simulink model "toneSelector"  (R2017b)
settings: Solver=VariableStepAuto  StartTime=0.0  StopTime=35  RelTol=1e-3
undefined symbols (not defined in the file): Ts
libraries: simulink x3, dspsnks4 x1
settings Model: Creator=pipe  LastModifiedBy=pipe

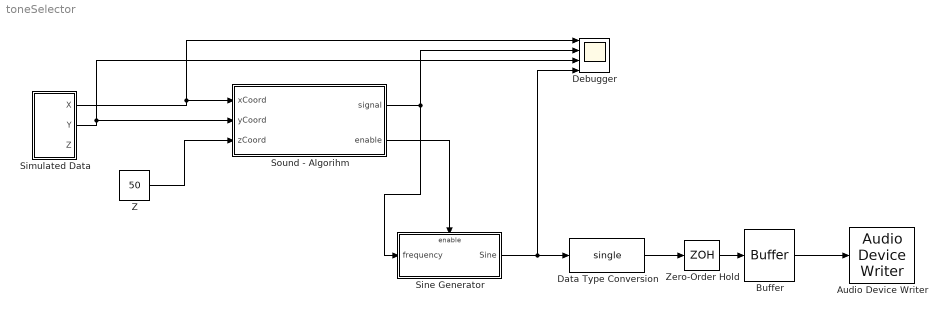
== system toneSelector ==
  Audio Device Writer : dspsnks4/Audio Device Writer  Driver=DirectSound  Device=Default  InheritSampleRate=on  SampleRate=40000  BitDepth=16-bit integer  BufferSize=4096  NumBuffers=10  DefaultOutputChannelMapping=on  OutputChannelMapping=1:2  OutputNumUnderrunSamples=off  DriverIdx=1  DeviceWarnFlag=''
  Buffer : Buffer  N=128  OutputFrames=off
  Data Type Conversion : DataTypeConversion  OutDataTypeStr=single
  "Debugger " : Scope  NumInputPorts=4
  Simulated Data : Subsystem
  Sine Generator : Subsystem  TreatAsAtomicUnit=on
  "Sound - Algorihm " : MATLAB Function  TreatAsAtomicUnit=on
  "Z " : Constant  Value=50  SampleTime=-1
  Zero-Order Hold : ZeroOrderHold  SampleTime=1/10000
  wires:
  "Sound - Algorihm "/1(signal) -> Sine Generator/1("frequency "), "Debugger "/2
  "Z "/1 -> "Sound - Algorihm "/3(zCoord)
  Simulated Data/1("X ") -> "Debugger "/1, "Sound - Algorihm "/1(xCoord)
  Simulated Data/2(Y) -> "Debugger "/3, "Sound - Algorihm "/2(yCoord)
  Sine Generator/1(Sine) -> "Debugger "/4, Data Type Conversion/1
  Buffer/1 -> Audio Device Writer/1
  Zero-Order Hold/1 -> Buffer/1
  Data Type Conversion/1 -> Zero-Order Hold/1
  "Sound - Algorihm "/2(enable) -> Sine Generator/Enable

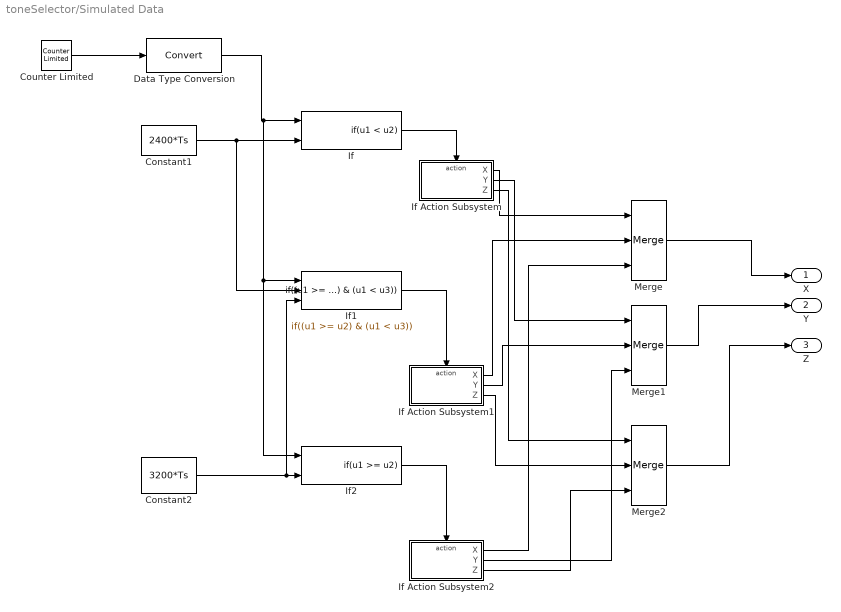
== system toneSelector/Simulated Data ==
  Constant1 : Constant  Value=2400*Ts  SampleTime=Ts
  Constant2 : Constant  Value=3200*Ts  SampleTime=Ts
  Counter Limited : simulink/Sources/Counter Limited  uplimit=3500  tsamp=Ts
  Data Type Conversion : DataTypeConversion
  If : If  NumInputs=2  IfExpression=u1 < u2  ShowElse=off
  If Action Subsystem : Subsystem  TreatAsAtomicUnit=on
  If Action Subsystem1 : Subsystem  TreatAsAtomicUnit=on
  If Action Subsystem2 : Subsystem  TreatAsAtomicUnit=on
  If1 : If  NumInputs=3  IfExpression=(u1 >= u2) & (u1 < u3)  ShowElse=off
  If2 : If  NumInputs=2  IfExpression=u1 >= u2  ShowElse=off
  Merge : Merge  Inputs=3
  Merge1 : Merge  Inputs=3
  Merge2 : Merge  Inputs=3
  "X " : Outport
  Y : Outport  Port=2
  "Z " : Outport  Port=3
  wires:
  If1/1 -> If Action Subsystem1/Action
  Constant2/1 -> If1/3, If2/2
  If Action Subsystem1/2(Y) -> Merge1/2
  If2/1 -> If Action Subsystem2/Action
  If/1 -> If Action Subsystem/Action
  Constant1/1 -> If1/2, If/2
  Data Type Conversion/1 -> If2/1, If1/1, If/1
  Counter Limited/1 -> Data Type Conversion/1
  Merge/1 -> "X "/1
  If Action Subsystem/1(X) -> Merge/1
  If Action Subsystem1/1(X) -> Merge/2
  If Action Subsystem2/1(X) -> Merge/3
  If Action Subsystem/2(Y) -> Merge1/1
  If Action Subsystem2/2(Y) -> Merge1/3
  If Action Subsystem/3("Z ") -> Merge2/1
  If Action Subsystem1/3("Z ") -> Merge2/2
  If Action Subsystem2/3("Z ") -> Merge2/3
  Merge2/1 -> "Z "/1
  Merge1/1 -> Y/1

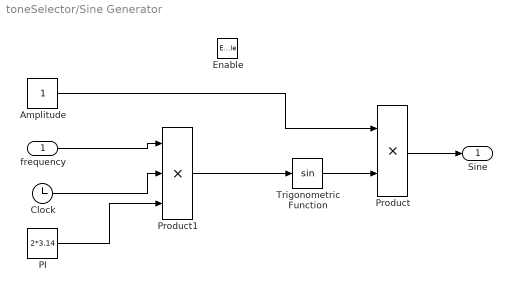
== system toneSelector/Sine Generator ==
  "frequency " : Inport
  Enable : EnablePort
  "Amplitude " : Constant
  Clock : Clock
  "PI " : Constant  Value=2*3.14
  Product : Product
  Product1 : Product  Inputs=3
  Trigonometric Function : Trigonometry
  Sine : Outport
  wires:
  Product/1 -> Sine/1
  Clock/1 -> Product1/2
  "Amplitude "/1 -> Product/1
  Trigonometric Function/1 -> Product/2
  "frequency "/1 -> Product1/1
  Product1/1 -> Trigonometric Function/1
  "PI "/1 -> Product1/3

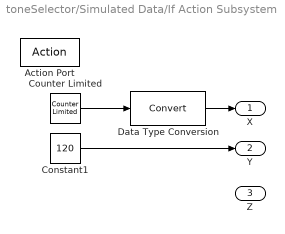
== system toneSelector/Simulated Data/If Action Subsystem ==
  Action Port : ActionPort  ActionType=then
  Constant1 : Constant  Value=120  SampleTime=Ts
  Counter Limited : simulink/Sources/Counter Limited  uplimit=255  tsamp=Ts
  Data Type Conversion : DataTypeConversion
  X : Outport  SampleTime=Ts  InitialOutput=[0]
  Y : Outport  Port=2  InitialOutput=[0]
  "Z " : Outport  Port=3
  wires:
  Constant1/1 -> Y/1
  Data Type Conversion/1 -> X/1
  Counter Limited/1 -> Data Type Conversion/1

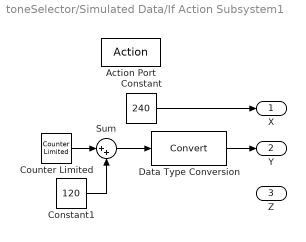
== system toneSelector/Simulated Data/If Action Subsystem1 ==
  Action Port : ActionPort  ActionType=then
  Constant : Constant  Value=240  SampleTime=Ts
  Constant1 : Constant  Value=120  SampleTime=Ts
  Counter Limited : simulink/Sources/Counter Limited  uplimit=255  tsamp=Ts
  Data Type Conversion : DataTypeConversion
  Sum : Sum  Inputs=|++
  X : Outport  InitialOutput=[0]
  Y : Outport  Port=2  InitialOutput=[0]
  "Z " : Outport  Port=3
  wires:
  Constant/1 -> X/1
  Data Type Conversion/1 -> Y/1
  Counter Limited/1 -> Sum/1
  Sum/1 -> Data Type Conversion/1
  Constant1/1 -> Sum/2

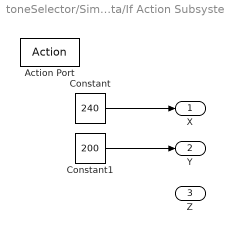
== system toneSelector/Simulated Data/If Action Subsystem2 ==
  Action Port : ActionPort  ActionType=then
  Constant : Constant  Value=240  SampleTime=Ts
  Constant1 : Constant  Value=200  SampleTime=Ts
  X : Outport  InitialOutput=[0]
  Y : Outport  Port=2  InitialOutput=[0]
  "Z " : Outport  Port=3
  wires:
  Constant1/1 -> Y/1
  Constant/1 -> X/1

== matlab function toneSelector/Sound - Algorihm  ==
  data: xCoord input; signal output; yCoord input; zCoord input; enable output
function [signal, enable]  = toneGenerator(xCoord,yCoord,zCoord)
%INFO

nBits = 8; % Number of bits for each coordinate

columns = 4; 
rows = 2; 
maxHeight = 100; %Key max Sensitivity height. Max Value = 2^nBits -1
enable = 0; 



actualQuadrant = zeros(rows,columns); 
xArrayLimits = zeros(columns +1); 
yArrayLimits = zeros(rows +1); 


for i = 1:(columns+1)
    xArrayLimits(i) = (i-1) * power(2,nBits)/columns; 
end


for i = (1:rows+1)
    yArrayLimits(i) = (i-1) * power(2,nBits)/rows; 
end
 

for i = 2:(columns+1)
    if (xCoord >= xArrayLimits(i-1)) && (xCoord < xArrayLimits(i))
        for j = 2:(rows +1)
            if (yCoord >= yArrayLimits(j-1)) && (yCoord < yArrayLimits(j))
                actualQuadrant((j-1),(i-1)) = 1; 
                break;
            end
        end
        break;
    end
end

pos = 0; 
pos = find(actualQuadrant == 1); % Position of "1" in matrix.  1 3 5 7
                                 %                             2 4 6 8                                 
signal = power(2,(pos(1)-1)/12) * 440; %400Hz base

if zCoord > maxHeight
    enable = 0; 
elseif zCoord <= maxHeight
    enable = 1; 
end


end
